simulink model "voltage_gain"  (R2024a)
settings: Solver=FixedStepDiscrete  StartTime=0.0  StopTime=100  RelTol=1e-3
settings Model: Creator=BVM  LastModifiedBy=BVM

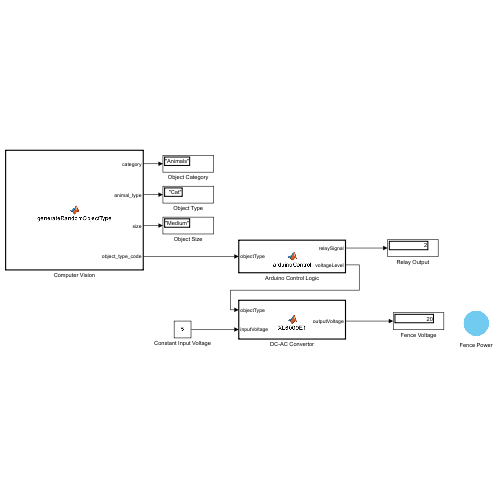
[thumbnail: Simulink's stored preview of the top-level diagram]
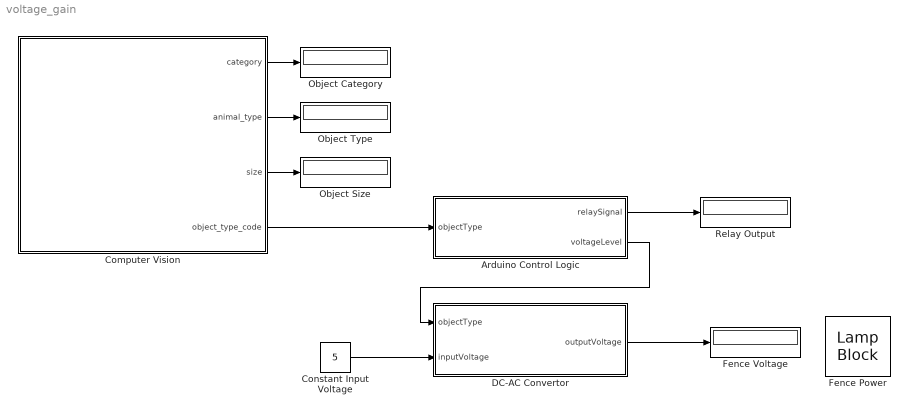
== system voltage_gain ==
  Arduino Control Logic : MATLAB Function  TreatAsAtomicUnit=on
  Computer Vision : MATLAB Function  TreatAsAtomicUnit=on
  Constant Input Voltage : Constant  Value=5
  DC-AC Convertor : MATLAB Function  TreatAsAtomicUnit=on
  Fence Power : LampBlock  LabelPosition=Hide  Icon=Circle
  Fence Voltage : Display
  Object Category : Display
  Object Size : Display
  Object Type : Display
  Relay Output : Display
  wires:
  DC-AC Convertor/1(outputVoltage) -> Fence Voltage/1
  Computer Vision/4(object_type_code) -> Arduino Control Logic/1(objectType)
  Arduino Control Logic/2(voltageLevel) -> DC-AC Convertor/1(objectType)
  Arduino Control Logic/1(relaySignal) -> Relay Output/1
  Computer Vision/1(category) -> Object Category/1
  Computer Vision/2(animal_type) -> Object Type/1
  Computer Vision/3(size) -> Object Size/1
  Constant Input Voltage/1 -> DC-AC Convertor/2(inputVoltage)

== matlab function voltage_gain/Arduino Control Logic ==
  data: objectType input; relaySignal output; voltageLevel output
function [relaySignal, voltageLevel] = arduinoControl(objectType)
% Simulate Arduino control logic based on detected object
% Input: objectType (1 = Human, 2 = Large Animal, 3 = Small Animal)
% Output: relaySignal (0 or 1), voltageLevel (0, 5, or 12)

    if objectType == 0
        relaySignal = 0; % Deactivate relay for human
        voltageLevel = 0; % No voltage
    elseif objectType == 1
        relaySignal = 1; % Activate relay
        voltageLevel = 1; % High voltage for large animals
    elseif objectType == 2
        relaySignal = 2; % Activate relay
        voltageLevel = 2; % Medium voltage for Medium animals
    else
        relaySignal = 3; % Activate relay
        voltageLevel = 3; % Lower voltage for small animals
    end
end

== matlab function voltage_gain/DC-AC Convertor ==
  data: objectType input; outputVoltage output; inputVoltage input
function outputVoltage  = XL6009E1(objectType, inputVoltage)
% XL6009E1 Simulates a DC-DC voltage regulator
% inputVoltage: the input voltage (constant 5V in this example)
% objectType: the type of detected object (1 = Human, 2 = Large Animal, 3 = Small Animal)
% outputVoltage: the regulated output voltage

    % Initialize output voltage
    outputVoltage = 0;
    
    
    % Determine the output voltage based on the detected object
    switch objectType
        case 0 % Human
            outputVoltage = 0;
       
        case 1 % Large Animal
            outputVoltage = 30;
            
        case 2 % Medium Animal
            outputVoltage = 20;
        case 3 % Small Animal
            outputVoltage = 10;
            
    end
end

== matlab function voltage_gain/Computer Vision ==
  data: category output string; animal_type output; size output; object_type_code output
function [category, animal_type,size,object_type_code]= generateRandomObjectType
% Define the data
data = {
    'Animals', 'Bison', 'Large', 1;
    'Animals', 'Boar', 'Large', 1;
    'Animals', 'Cow', 'Large', 1;
    'Animals', 'Coyote', 'Large', 1;
    'Animals', 'Deer', 'Large', 1;
    'Animals', 'Elephant', 'Large', 1;
    'Animals', 'Gorilla', 'Large', 1;
    'Animals', 'Hippopotamus', 'Large', 1;
    'Animals', 'Horse', 'Large', 1;
    'Animals', 'Human', 'Large', 1;
    'Animals', 'Leopard', 'Large', 1;
    'Animals', 'Lion', 'Large', 1;
    'Animals', 'Okapi', 'Large', 1;
    'Animals', 'Orangutan', 'Large', 1;
    'Human', 'Human', 'small', 0;
    'Human', 'Human', 'small', 0;
    'Human', 'Human', 'small', 0;
    'Human', 'Human', 'small', 0;
    'Human', 'Human', 'small', 0;
    'Human', 'Human', 'small', 0;
    'Human', 'Human', 'small', 0;
    'Animals', 'Ox', 'Large', 1;
    'Animals', 'Panda', 'Large', 1;
    'Animals', 'Reindeer', 'Large', 1;
    'Animals', 'Rhinoceros', 'Large', 1;
    'Animals', 'Tiger', 'Large', 1;
    'Animals', 'Wolf', 'Large', 1;
    'Birds', 'None', 'Large', 1;
    'Reptiles', 'None', 'Large', 1;
    'Insects', 'None', 'Large', 1;
    'Marine Animals', 'Shark', 'Large', 1;
    'Marine Animals', 'Whale', 'Large', 1;
    'Animals', 'Boar', 'Medium', 2;
    'Animals', 'Cat', 'Medium', 2;
    'Animals', 'Chimpanzee', 'Medium', 2;
    'Animals', 'Dog', 'Medium', 2;
    'Animals', 'Dolphin', 'Medium', 2;
    'Animals', 'Donkey', 'Medium', 2;
    'Animals', 'Fox', 'Medium', 2;
    'Animals', 'Goat', 'Medium', 2;
    'Animals', 'Hare', 'Medium', 2;
    'Animals', 'Hedgehog', 'Medium', 2;
    'Animals', 'Hyena', 'Medium', 2;
    'Animals', 'Kangaroo', 'Medium', 2;
    'Animals', 'Koala', 'Medium', 2;
    'Animals', 'Leopard', 'Medium', 2;
    'Animals', 'Pig', 'Medium', 2;
    'Animals', 'Turkey', 'Medium', 2;
    'Animals', 'Wombat', 'Medium', 2;
    'Animals', 'Possum', 'Medium', 2;
    'Animals', 'Raccoon', 'Medium', 2;
    'Animals', 'Porcupine', 'Medium', 2;
    'Birds', 'Eagle', 'Medium', 2;
    'Birds', 'Fire', 'Medium', 2;
    'Birds', 'Flamingo', 'Medium', 2;
    'Birds', 'Penguin', 'Medium', 2;
    'Animals', 'Zebra', 'Medium', 2;
    'Reptiles', 'None', 'Medium', 2;
    'Insects', 'None', 'Medium', 2;
    'Marine Animals', 'None', 'Medium', 2;
    'Animals', 'Cat', 'Small', 3;
    'Animals', 'Hamster', 'Small', 3;
    'Animals', 'Hedgehog', 'Small', 3;
    'Animals', 'Jellyfish', 'Small', 3;
    'Animals', 'Ladybugs', 'Small', 3;
    'Animals', 'Mouse', 'Small', 3;
    'Animals', 'Otter', 'Small', 3;
    'Animals', 'Oyster', 'Small', 3;
    'Animals', 'Porcupine', 'Small', 3;
    'Animals', 'Possum', 'Small', 3;
    'Animals', 'Raccoon', 'Small', 3;
    'Animals', 'Rat', 'Small', 3;
    'Animals', 'Seahorse', 'Small', 3;
    'Animals', 'Squirrel', 'Small', 3;
    'Animals', 'Starfish', 'Small', 3;
    'Birds', 'Crow', 'Small', 3;
    'Birds', 'Duck', 'Small', 3;
    'Birds', 'Goose', 'Small', 3;
    'Birds', 'Hornbill', 'Small', 3;
    'Birds', 'Hummingbird', 'Small', 3;
    'Birds', 'Owl', 'Small', 3;
    'Birds', 'Parrot', 'Small', 3;
    'Birds', 'Pigeon', 'Small', 3;
    'Birds', 'Sandpiper', 'Small', 3;
    'Birds', 'Sparrow', 'Small', 3;
    'Birds', 'Swan', 'Small', 3;
    'Birds', 'Woodpecker', 'Small', 3;
    'Reptiles', 'Lizard', 'Small', 3;
    'Reptiles', 'Snake', 'Small', 3;
    'Insects', 'Bee', 'Small', 3;
    'Insects', 'Beetle', 'Small', 3;
    'Insects', 'Butterfly', 'Small', 3;
    'Insects', 'Caterpillar', 'Small', 3;
    'Insects', 'Cockroach', 'Small', 3;
    'Insects', 'Fly', 'Small', 3;
    'Insects', 'Grasshopper', 'Small', 3;
    'Insects', 'Mosquito', 'Small', 3;
    'Insects', 'Moth', 'Small', 3;
    'Marine Animals', 'Crab', 'Small', 3;
    'Marine Animals', 'Goldfish', 'Small', 3;
    'Marine Animals', 'Lobster', 'Small', 3;
    'Marine Animals', 'Octopus', 'Small', 3;
    'Marine Animals', 'Squid', 'Small', 3;
    'Human', 'Human', 'small', 0;
};

% Convert to table
data_table = cell2table(data, 'VariableNames', {'Category', 'AnimalType', 'Size', 'Code'});

category = "";
animal_type = "";
size="";

% Randomly select a row and get the Code
random_row = data_table(randi(height(data_table)), :);
object_type_code = random_row.Code;
category_1=random_row.Category;
category = string(category_1);
animal_type_1=random_row.AnimalType;
animal_type=string(animal_type_1);
size_1=random_row.Size;
size=string(size_1);
